simulink model "fir_32tap_8cores"  (R2019b)
settings: Solver=VariableStepAuto  StartTime=0.0  StopTime=T/2  RelTol=1e-3
InitFcn:
  | xmcCheckSlxPath(bdroot)
  | setup
StopFcn:
  | %compare
values from neighbouring files (symbols this model uses):
  c = [30 31 28 29 26 27 24 25 22 23 20 21 18 19 16 17      14 15 12 13 10 11 8 9 6 7 4 5 2 3 0 1]    [setup.m]
undefined symbols (not defined in the file or in its folder): xc7vx485tffg1157
libraries: dspsrcs4 x15, ModelComposer x10, dspsigops x4
settings Model: Creator=abehbood  LastModifiedBy=abehbood
settings SFSimCC: CustomCodeUndefinedFunction=UseInterfaceOnly

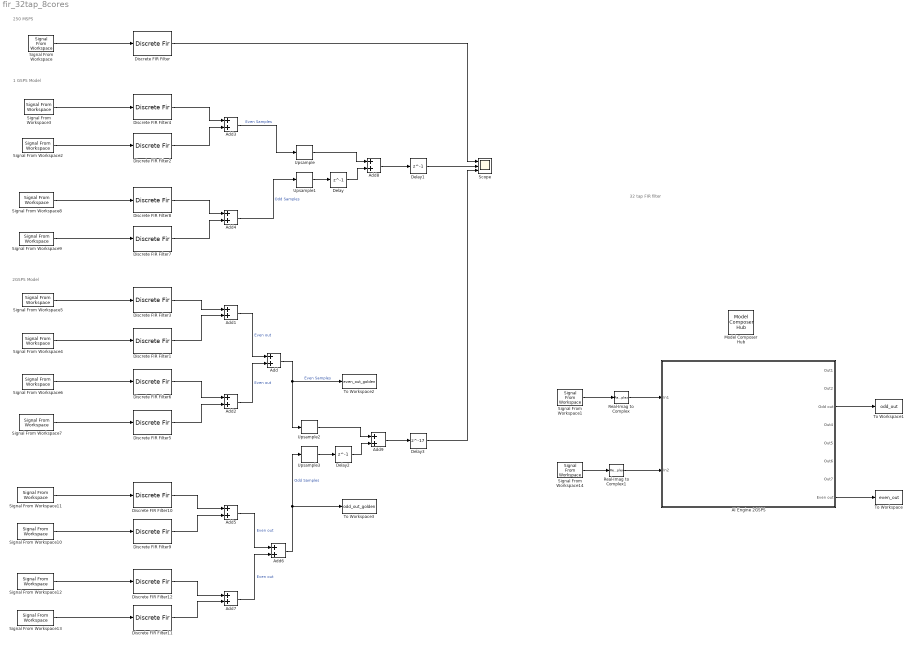
== system fir_32tap_8cores ==
  note: 32 tap FIR filter
  note: 250 MSPS
  note: 2GSPS Model
  note: 1 GSPS Model
  AI Engine 2GSPS : Subsystem
  Add{,1..9} (10 alike) : Sum
  Delay : Delay  DelayLength=1
  Delay1 : Delay  DelayLength=1
  Delay2 : Delay  DelayLength=1
  Delay3 : Delay  DelayLength=17
  Discrete FIR Filter : DiscreteFir  Coefficients=c  InputProcessing=Columns as channels (frame based)  CoefDataTypeStr=int16  ProductDataTypeStr=fixdt(1,48,0)  AccumDataTypeStr=fixdt(1,48,0)  OutDataTypeStr=int16
  Discrete FIR Filter1 : DiscreteFir  Coefficients=c(1:2:32/2)  InputProcessing=Columns as channels (frame based)  CoefDataTypeStr=int16  OutDataTypeStr=int16
  Discrete FIR Filter10 : DiscreteFir  Coefficients=c(32/2+1:2:end)  InputProcessing=Columns as channels (frame based)  CoefDataTypeStr=int16  OutDataTypeStr=int16
  Discrete FIR Filter11 : DiscreteFir  Coefficients=c(2:2:32/2)  InputProcessing=Columns as channels (frame based)  CoefDataTypeStr=int16  OutDataTypeStr=int16
  Discrete FIR Filter12 : DiscreteFir  Coefficients=c(32/2+2:2:end)  InputProcessing=Columns as channels (frame based)  CoefDataTypeStr=int16  OutDataTypeStr=int16
  Discrete FIR Filter2 : DiscreteFir  Coefficients=c(2:2:end)  InputProcessing=Columns as channels (frame based)  CoefDataTypeStr=int16  OutDataTypeStr=int16
  Discrete FIR Filter3 : DiscreteFir  Coefficients=c(32/2+1:2:end)  InputProcessing=Columns as channels (frame based)  CoefDataTypeStr=int16  OutDataTypeStr=int16
  Discrete FIR Filter4 : DiscreteFir  Coefficients=c(1:2:end)  InputProcessing=Columns as channels (frame based)  CoefDataTypeStr=int16  OutDataTypeStr=int16
  Discrete FIR Filter5 : DiscreteFir  Coefficients=c(2:2:32/2)  InputProcessing=Columns as channels (frame based)  CoefDataTypeStr=int16  OutDataTypeStr=int16
  Discrete FIR Filter6 : DiscreteFir  Coefficients=c(32/2+2:2:end)  InputProcessing=Columns as channels (frame based)  CoefDataTypeStr=int16  OutDataTypeStr=int16
  Discrete FIR Filter7 : DiscreteFir  Coefficients=c(2:2:end)  InputProcessing=Columns as channels (frame based)  CoefDataTypeStr=int16  OutDataTypeStr=int16
  Discrete FIR Filter8 : DiscreteFir  Coefficients=c(1:2:end)  InputProcessing=Columns as channels (frame based)  CoefDataTypeStr=int16  OutDataTypeStr=int16
  Discrete FIR Filter9 : DiscreteFir  Coefficients=c(1:2:32/2)  InputProcessing=Columns as channels (frame based)  CoefDataTypeStr=int16  OutDataTypeStr=int16
  Model Composer Hub : ModelComposer/Model Composer Hub  CodeGeneration=off  TargetDirectory=./code  SubsystemName=AI Engine 2GSPS  ExportType=AI Engines  IpVendor=xilinx.com  IpLibrary=hls  IpVersion=1.0  IpHWLanguage=Verilog  CreateTestbench=on  TestbenchStackSize=10  AieCompilerOptions={}  RunAieSim=on  LaunchVitisAnalyzer=off  AieSimTimeout=50000  RunX86Sim=off  X86SimTimeout=10  ProjDevice=xc7vx485tffg1157-1  ProjDevicePart=xc7vx485tffg1157-1  SamplePeriod=-1  ClockFrequency=200  DataPathParallelism=1
  Real-Imag to Complex : RealImagToComplex  Input=Real
  Real-Imag to Complex1 : RealImagToComplex  Input=Real
  Scope : Scope  NumInputPorts=3
  Signal From Workspace : dspsrcs4/Signal From Workspace  X=in  Ts=.5  nsamps=1  OutputAfterFinalValue=Setting to zero  ignoreOrWarnInputAndFrameLengths=off  OutputFrames=off
  Signal From Workspace{1,3,5,9,12} (5 alike) : dspsrcs4/Signal From Workspace  X=in_odd  Ts=1  nsamps=1  OutputAfterFinalValue=Setting to zero  ignoreOrWarnInputAndFrameLengths=off  OutputFrames=off
  Signal From Workspace10 : dspsrcs4/Signal From Workspace  X=in_even_skip_9  Ts=1  nsamps=1  OutputAfterFinalValue=Setting to zero  ignoreOrWarnInputAndFrameLengths=off  OutputFrames=off
  Signal From Workspace11 : dspsrcs4/Signal From Workspace  X=in_even_skip_1  Ts=1  nsamps=1  OutputAfterFinalValue=Setting to zero  ignoreOrWarnInputAndFrameLengths=off  OutputFrames=off
  Signal From Workspace13 : dspsrcs4/Signal From Workspace  X=in_odd_skip_8  Ts=1  nsamps=1  OutputAfterFinalValue=Setting to zero  ignoreOrWarnInputAndFrameLengths=off  OutputFrames=off
  Signal From Workspace14 : dspsrcs4/Signal From Workspace  X=in_even  Ts=1  nsamps=1  OutputAfterFinalValue=Setting to zero  ignoreOrWarnInputAndFrameLengths=off  OutputFrames=off
  Signal From Workspace2 : dspsrcs4/Signal From Workspace  X=in_even  Ts=1  nsamps=1  OutputAfterFinalValue=Setting to zero  ignoreOrWarnInputAndFrameLengths=off  OutputFrames=off
  Signal From Workspace4 : dspsrcs4/Signal From Workspace  X=in_odd_skip_8  Ts=1  nsamps=1  OutputAfterFinalValue=Setting to zero  ignoreOrWarnInputAndFrameLengths=off  OutputFrames=off
  Signal From Workspace6 : dspsrcs4/Signal From Workspace  X=in_even  Ts=1  nsamps=1  OutputAfterFinalValue=Setting to zero  ignoreOrWarnInputAndFrameLengths=off  OutputFrames=off
  Signal From Workspace7 : dspsrcs4/Signal From Workspace  X=in_even_skip_8  Ts=1  nsamps=1  OutputAfterFinalValue=Setting to zero  ignoreOrWarnInputAndFrameLengths=off  OutputFrames=off
  Signal From Workspace8 : dspsrcs4/Signal From Workspace  X=in_even_skip_1  Ts=1  nsamps=1  OutputAfterFinalValue=Setting to zero  ignoreOrWarnInputAndFrameLengths=off  OutputFrames=off
  To Workspace : ToWorkspace  VariableName=even_out  SaveFormat=Structure  SampleTime=-1
  To Workspace1 : ToWorkspace  VariableName=odd_out  SaveFormat=Structure  SampleTime=-1
  To Workspace2 : ToWorkspace  VariableName=even_out_golden  SampleTime=-1
  To Workspace3 : ToWorkspace  VariableName=odd_out_golden  SampleTime=-1
  Upsample{,1..3} (4 alike) : dspsigops/Upsample  N=2  phase=0  InputProcessing=Columns as channels (frame based)  RateOptions=Allow multirate processing  ic=0  mode=Unused parameter value
  wires:
  Signal From Workspace3/1 -> Discrete FIR Filter4/1
  Signal From Workspace2/1 -> Discrete FIR Filter2/1
  Add1/1 -> Add/1  "Even out"
  Discrete FIR Filter4/1 -> Add3/1
  Signal From Workspace4/1 -> Discrete FIR Filter1/1
  Signal From Workspace5/1 -> Discrete FIR Filter3/1
  Signal From Workspace6/1 -> Discrete FIR Filter6/1
  Signal From Workspace7/1 -> Discrete FIR Filter5/1
  Discrete FIR Filter5/1 -> Add2/2
  Discrete FIR Filter6/1 -> Add2/1
  Add2/1 -> Add/2  "Even out"
  Discrete FIR Filter2/1 -> Add3/2
  Add3/1 -> Upsample/1  "Even Samples"
  Discrete FIR Filter8/1 -> Add4/1
  Add4/1 -> Upsample1/1  "Odd Samples"
  Discrete FIR Filter7/1 -> Add4/2
  Signal From Workspace8/1 -> Discrete FIR Filter8/1
  Signal From Workspace9/1 -> Discrete FIR Filter7/1
  Discrete FIR Filter12/1 -> Add7/1
  Signal From Workspace12/1 -> Discrete FIR Filter12/1
  Discrete FIR Filter11/1 -> Add7/2
  Add5/1 -> Add6/1  "Even out"
  Signal From Workspace13/1 -> Discrete FIR Filter11/1
  Discrete FIR Filter9/1 -> Add5/2
  Signal From Workspace10/1 -> Discrete FIR Filter9/1
  Add7/1 -> Add6/2  "Even out"
  Signal From Workspace11/1 -> Discrete FIR Filter10/1
  Discrete FIR Filter10/1 -> Add5/1
  Discrete FIR Filter3/1 -> Add1/1
  Discrete FIR Filter1/1 -> Add1/2
  Upsample1/1 -> Delay/1
  Upsample/1 -> Add8/1
  Delay/1 -> Add8/2
  Add8/1 -> Delay1/1
  Delay1/1 -> Scope/2
  Upsample3/1 -> Delay2/1
  Add6/1 -> To Workspace3/1, Upsample3/1  "Odd Samples"
  Upsample2/1 -> Add9/1
  Delay2/1 -> Add9/2
  Add/1 -> To Workspace2/1, Upsample2/1  "Even Samples"
  Discrete FIR Filter/1 -> Scope/1
  Add9/1 -> Delay3/1
  Delay3/1 -> Scope/3
  Signal From Workspace/1 -> Discrete FIR Filter/1
  Signal From Workspace1/1 -> Real-Imag to Complex/1
  Signal From Workspace14/1 -> Real-Imag to Complex1/1
  Real-Imag to Complex/1 -> AI Engine 2GSPS/1(In1)
  Real-Imag to Complex1/1 -> AI Engine 2GSPS/2(In2)
  AI Engine 2GSPS/8(Even out) -> To Workspace/1
  AI Engine 2GSPS/3(Odd out) -> To Workspace1/1

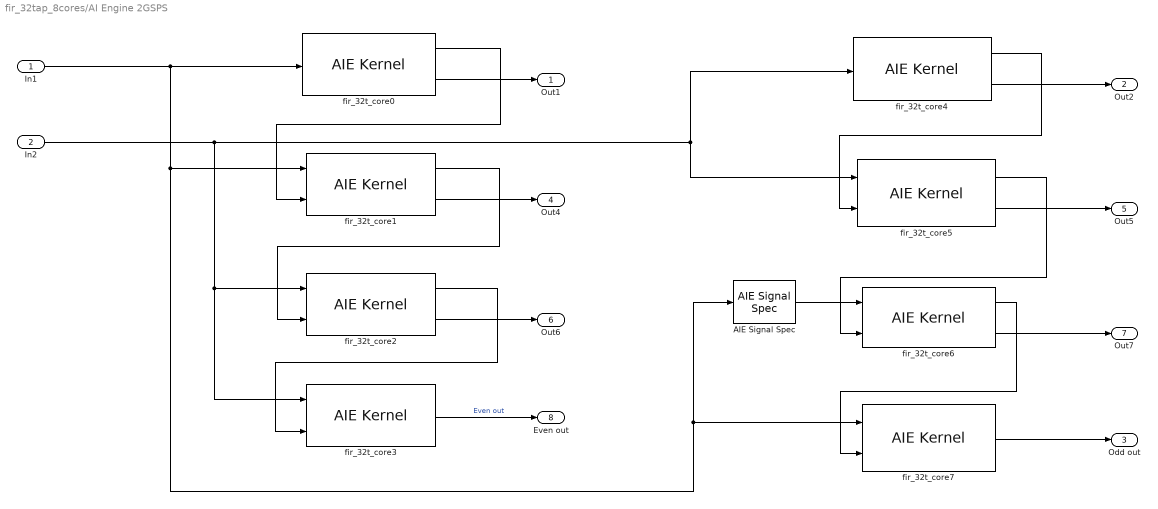
== system fir_32tap_8cores/AI Engine 2GSPS ==
  In1 : Inport
  In2 : Inport  Port=2
  AIE Signal Spec : ModelComposer/AIE Signal Spec  DestFifoDepth=1  SrcFifoDepth=0  PlioWidth=NA
  fir_32t_core0 : ModelComposer/AIE Kernel  PortAttributesTable={'Input', 'sig_in', 'input_stream_cint16 *', '', '', '', '';'Output', 'cascadeout', 'output_stream_cacc48 *', '', '', '', '1';'Output', 'data_out', 'output_stream_cint16 *', '', '', '', '1'}  PortAttributesEnablement={'off', 'off', 'off', 'off', 'off', 'off', 'off';'off', 'off', 'off', 'off', 'off', 'off', 'on';'off', 'off', 'off', 'off', 'off', 'off', 'on'}  FormalArgDecls={'input_stream_cint16 * sig_in', 'output_stream_cacc48 * cascadeout', 'output_stream_cint16 * data_out'}  PortWindowSizes={0.000000000000000000e+00, 0.000000000000000000e+00, 0.000000000000000000e+00}  PortWindowMargins={0.000000000000000000e+00, 0.000000000000000000e+00, 0.000000000000000000e+00}  PortSynchronicities={'sync', 'sync', 'sync'}  PortSignalSizes={0.000000000000000000e+00, 1.000000000000000000e+00, 1.000000000000000000e+00}  SimLibPath=''  FunctionTabVisible=on  FunctionDescription=void fir_32t_core0(input_stream_cint16 * sig_in, output_stream_cacc48 * cascadeout, output_stream_cint16 * data_out)  KernelHeaderFile=src/kernels/inc/fir_32t_core0.h  KernelFunction=fir_32t_core0  KernelFunctionSelect=<empty>  KernelInitFunction=fir_32t_core0_init  KernelSourceFile=fir_32t_core0.cc  KernelSearchPaths={'./data', './src', './src/include', './src/kernels/inc', './src/kernels/src_template'}  PreProcOptions={}  CoreRuntimeRatio=0.9
  fir_32t_core1 : ModelComposer/AIE Kernel  PortAttributesTable={'Input', 'sign_in', 'input_stream_cint16 *', '', '', '', '';'Input', 'cascadein', 'input_stream_cacc48 *', '', '', '', '';'Output', 'cascadeout', 'output_stream_cacc48 *', '', '', '', '1';'Output', 'data_out', 'output_stream_cint16 *', '', '', '', '1'}  PortAttributesEnablement={'off', 'off', 'off', 'off', 'off', 'off', 'off';'off', 'off', 'off', 'off', 'off', 'off', 'off';'off', 'off', 'off', 'off', 'off', 'off', 'on';'off', 'off', 'off', 'off', 'off', 'off', 'on'}  FormalArgDecls={'input_stream_cint16 * sign_in', 'input_stream_cacc48 * cascadein', 'output_stream_cacc48 * cascadeout', 'output_stream_cint16 * data_out'}  PortWindowSizes={0.000000000000000000e+00, 0.000000000000000000e+00, 0.000000000000000000e+00, 0.000000000000000000e+00}  PortWindowMargins={0.000000000000000000e+00, 0.000000000000000000e+00, 0.000000000000000000e+00, 0.000000000000000000e+00}  PortSynchronicities={'sync', 'sync', 'sync', 'sync'}  PortSignalSizes={0.000000000000000000e+00, 0.000000000000000000e+00, 1.000000000000000000e+00, 1.000000000000000000e+00}  SimLibPath=''  FunctionTabVisible=on  FunctionDescription=void fir_32t_core1(input_stream_cint16 * sign_in, input_stream_cacc48 * cascadein, output_stream_cacc48 * cascadeout, output_stream_cint16 * data_out)  KernelHeaderFile=src/kernels/inc/fir_32t_core1.h  KernelFunction=fir_32t_core1  KernelFunctionSelect=<empty>  KernelInitFunction=fir_32t_core1_init  KernelSourceFile=fir_32t_core1.cc  KernelSearchPaths={'./data', './src', './src/include', './src/kernels/inc', './src/kernels/src_template'}  PreProcOptions={}  CoreRuntimeRatio=0.9
  fir_32t_core2 : ModelComposer/AIE Kernel  PortAttributesTable={'Input', 'sign_in', 'input_stream_cint16 *', '', '', '', '';'Input', 'cascadein', 'input_stream_cacc48 *', '', '', '', '';'Output', 'cascadeout', 'output_stream_cacc48 *', '', '', '', '1';'Output', 'data_out', 'output_stream_cint16 *', '', '', '', '1'}  PortAttributesEnablement={'off', 'off', 'off', 'off', 'off', 'off', 'off';'off', 'off', 'off', 'off', 'off', 'off', 'off';'off', 'off', 'off', 'off', 'off', 'off', 'on';'off', 'off', 'off', 'off', 'off', 'off', 'on'}  FormalArgDecls={'input_stream_cint16 * sign_in', 'input_stream_cacc48 * cascadein', 'output_stream_cacc48 * cascadeout', 'output_stream_cint16 * data_out'}  PortWindowSizes={0.000000000000000000e+00, 0.000000000000000000e+00, 0.000000000000000000e+00, 0.000000000000000000e+00}  PortWindowMargins={0.000000000000000000e+00, 0.000000000000000000e+00, 0.000000000000000000e+00, 0.000000000000000000e+00}  PortSynchronicities={'sync', 'sync', 'sync', 'sync'}  PortSignalSizes={0.000000000000000000e+00, 0.000000000000000000e+00, 1.000000000000000000e+00, 1.000000000000000000e+00}  SimLibPath=''  FunctionTabVisible=on  FunctionDescription=void fir_32t_core2(input_stream_cint16 * sign_in, input_stream_cacc48 * cascadein, output_stream_cacc48 * cascadeout, output_stream_cint16 * data_out)  KernelHeaderFile=src/kernels/inc/fir_32t_core2.h  KernelFunction=fir_32t_core2  KernelFunctionSelect=<empty>  KernelInitFunction=fir_32t_core2_init  KernelSourceFile=fir_32t_core2.cc  KernelSearchPaths={'./data', './src', './src/include', './src/kernels/inc', './src/kernels/src_template'}  PreProcOptions={}  CoreRuntimeRatio=0.9
  fir_32t_core3 : ModelComposer/AIE Kernel  PortAttributesTable={'Input', 'sign_in', 'input_stream_cint16 *', '', '', '', '';'Input', 'cascadein', 'input_stream_cacc48 *', '', '', '', '';'Output', 'data_out', 'output_stream_cint16 *', '', '', '', '1'}  PortAttributesEnablement={'off', 'off', 'off', 'off', 'off', 'off', 'off';'off', 'off', 'off', 'off', 'off', 'off', 'off';'off', 'off', 'off', 'off', 'off', 'off', 'on'}  FormalArgDecls={'input_stream_cint16 * sign_in', 'input_stream_cacc48 * cascadein', 'output_stream_cint16 * data_out'}  PortWindowSizes={0.000000000000000000e+00, 0.000000000000000000e+00, 0.000000000000000000e+00}  PortWindowMargins={0.000000000000000000e+00, 0.000000000000000000e+00, 0.000000000000000000e+00}  PortSynchronicities={'sync', 'sync', 'sync'}  PortSignalSizes={0.000000000000000000e+00, 0.000000000000000000e+00, 1.000000000000000000e+00}  SimLibPath=''  FunctionTabVisible=on  FunctionDescription=void fir_32t_core3(input_stream_cint16 * sign_in, input_stream_cacc48 * cascadein, output_stream_cint16 * data_out)  KernelHeaderFile=src/kernels/inc/fir_32t_core3.h  KernelFunction=fir_32t_core3  KernelFunctionSelect=<empty>  KernelInitFunction=fir_32t_core3_init  KernelSourceFile=fir_32t_core3.cc  KernelSearchPaths={'./data', './src', './src/include', './src/kernels/inc', './src/kernels/src_template'}  PreProcOptions={}  CoreRuntimeRatio=0.9
  fir_32t_core4 : ModelComposer/AIE Kernel  PortAttributesTable={'Input', 'sig_in', 'input_stream_cint16 *', '', '', '', '';'Output', 'cascadeout', 'output_stream_cacc48 *', '', '', '', '1';'Output', 'data_out', 'output_stream_cint16 *', '', '', '', '1'}  PortAttributesEnablement={'off', 'off', 'off', 'off', 'off', 'off', 'off';'off', 'off', 'off', 'off', 'off', 'off', 'on';'off', 'off', 'off', 'off', 'off', 'off', 'on'}  FormalArgDecls={'input_stream_cint16 * sig_in', 'output_stream_cacc48 * cascadeout', 'output_stream_cint16 * data_out'}  PortWindowSizes={0.000000000000000000e+00, 0.000000000000000000e+00, 0.000000000000000000e+00}  PortWindowMargins={0.000000000000000000e+00, 0.000000000000000000e+00, 0.000000000000000000e+00}  PortSynchronicities={'sync', 'sync', 'sync'}  PortSignalSizes={0.000000000000000000e+00, 1.000000000000000000e+00, 1.000000000000000000e+00}  SimLibPath=''  FunctionTabVisible=on  FunctionDescription=void fir_32t_core4(input_stream_cint16 * sig_in, output_stream_cacc48 * cascadeout, output_stream_cint16 * data_out)  KernelHeaderFile=src/kernels/inc/fir_32t_core4.h  KernelFunction=fir_32t_core4  KernelFunctionSelect=<empty>  KernelInitFunction=fir_32t_core4_init  KernelSourceFile=fir_32t_core4.cc  KernelSearchPaths={'./data', './src', './src/include', './src/kernels/inc', './src/kernels/src_template'}  PreProcOptions={}  CoreRuntimeRatio=0.9
  fir_32t_core5 : ModelComposer/AIE Kernel  PortAttributesTable={'Input', 'sign_in', 'input_stream_cint16 *', '', '', '', '';'Input', 'cascadein', 'input_stream_cacc48 *', '', '', '', '';'Output', 'cascadeout', 'output_stream_cacc48 *', '', '', '', '1';'Output', 'data_out', 'output_stream_cint16 *', '', '', '', '1'}  PortAttributesEnablement={'off', 'off', 'off', 'off', 'off', 'off', 'off';'off', 'off', 'off', 'off', 'off', 'off', 'off';'off', 'off', 'off', 'off', 'off', 'off', 'on';'off', 'off', 'off', 'off', 'off', 'off', 'on'}  FormalArgDecls={'input_stream_cint16 * sign_in', 'input_stream_cacc48 * cascadein', 'output_stream_cacc48 * cascadeout', 'output_stream_cint16 * data_out'}  PortWindowSizes={0.000000000000000000e+00, 0.000000000000000000e+00, 0.000000000000000000e+00, 0.000000000000000000e+00}  PortWindowMargins={0.000000000000000000e+00, 0.000000000000000000e+00, 0.000000000000000000e+00, 0.000000000000000000e+00}  PortSynchronicities={'sync', 'sync', 'sync', 'sync'}  PortSignalSizes={0.000000000000000000e+00, 0.000000000000000000e+00, 1.000000000000000000e+00, 1.000000000000000000e+00}  SimLibPath=''  FunctionTabVisible=on  FunctionDescription=void fir_32t_core5(input_stream_cint16 * sign_in, input_stream_cacc48 * cascadein, output_stream_cacc48 * cascadeout, output_stream_cint16 * data_out)  KernelHeaderFile=src/kernels/inc/fir_32t_core5.h  KernelFunction=fir_32t_core5  KernelFunctionSelect=<empty>  KernelInitFunction=fir_32t_core5_init  KernelSourceFile=fir_32t_core5.cc  KernelSearchPaths={'./data', './src', './src/include', './src/kernels/inc', './src/kernels/src_template'}  PreProcOptions={}  CoreRuntimeRatio=0.9
  fir_32t_core6 : ModelComposer/AIE Kernel  PortAttributesTable={'Input', 'sign_in', 'input_stream_cint16 *', '', '', '', '';'Input', 'cascadein', 'input_stream_cacc48 *', '', '', '', '';'Output', 'cascadeout', 'output_stream_cacc48 *', '', '', '', '1';'Output', 'data_out', 'output_stream_cint16 *', '', '', '', '1'}  PortAttributesEnablement={'off', 'off', 'off', 'off', 'off', 'off', 'off';'off', 'off', 'off', 'off', 'off', 'off', 'off';'off', 'off', 'off', 'off', 'off', 'off', 'on';'off', 'off', 'off', 'off', 'off', 'off', 'on'}  FormalArgDecls={'input_stream_cint16 * sign_in', 'input_stream_cacc48 * cascadein', 'output_stream_cacc48 * cascadeout', 'output_stream_cint16 * data_out'}  PortWindowSizes={0.000000000000000000e+00, 0.000000000000000000e+00, 0.000000000000000000e+00, 0.000000000000000000e+00}  PortWindowMargins={0.000000000000000000e+00, 0.000000000000000000e+00, 0.000000000000000000e+00, 0.000000000000000000e+00}  PortSynchronicities={'sync', 'sync', 'sync', 'sync'}  PortSignalSizes={0.000000000000000000e+00, 0.000000000000000000e+00, 1.000000000000000000e+00, 1.000000000000000000e+00}  SimLibPath=''  FunctionTabVisible=on  FunctionDescription=void fir_32t_core6(input_stream_cint16 * sign_in, input_stream_cacc48 * cascadein, output_stream_cacc48 * cascadeout, output_stream_cint16 * data_out)  KernelHeaderFile=src/kernels/inc/fir_32t_core6.h  KernelFunction=fir_32t_core6  KernelFunctionSelect=<empty>  KernelInitFunction=fir_32t_core6_init  KernelSourceFile=fir_32t_core6.cc  KernelSearchPaths={'./data', './src', './src/include', './src/kernels/inc', './src/kernels/src_template'}  PreProcOptions={}  CoreRuntimeRatio=0.9
  fir_32t_core7 : ModelComposer/AIE Kernel  PortAttributesTable={'Input', 'sign_in', 'input_stream_cint16 *', '', '', '', '';'Input', 'cascadein', 'input_stream_cacc48 *', '', '', '', '';'Output', 'data_out', 'output_stream_cint16 *', '', '', '', '1'}  PortAttributesEnablement={'off', 'off', 'off', 'off', 'off', 'off', 'off';'off', 'off', 'off', 'off', 'off', 'off', 'off';'off', 'off', 'off', 'off', 'off', 'off', 'on'}  FormalArgDecls={'input_stream_cint16 * sign_in', 'input_stream_cacc48 * cascadein', 'output_stream_cint16 * data_out'}  PortWindowSizes={0.000000000000000000e+00, 0.000000000000000000e+00, 0.000000000000000000e+00}  PortWindowMargins={0.000000000000000000e+00, 0.000000000000000000e+00, 0.000000000000000000e+00}  PortSynchronicities={'sync', 'sync', 'sync'}  PortSignalSizes={0.000000000000000000e+00, 0.000000000000000000e+00, 1.000000000000000000e+00}  SimLibPath=''  FunctionTabVisible=on  FunctionDescription=void fir_32t_core7(input_stream_cint16 * sign_in, input_stream_cacc48 * cascadein, output_stream_cint16 * data_out)  KernelHeaderFile=src/kernels/inc/fir_32t_core7.h  KernelFunction=fir_32t_core7  KernelFunctionSelect=<empty>  KernelInitFunction=fir_32t_core7_init  KernelSourceFile=fir_32t_core7.cc  KernelSearchPaths={'./data', './src', './src/include', './src/kernels/inc', './src/kernels/src_template'}  PreProcOptions={}  CoreRuntimeRatio=0.9
  Out1 : Outport  VectorParamsAs1DForOutWhenUnconnected=off
  Out2 : Outport  Port=2  VectorParamsAs1DForOutWhenUnconnected=off
  Odd out : Outport  Port=3  VectorParamsAs1DForOutWhenUnconnected=off
  Out4 : Outport  Port=4  VectorParamsAs1DForOutWhenUnconnected=off
  Out5 : Outport  Port=5  VectorParamsAs1DForOutWhenUnconnected=off
  Out6 : Outport  Port=6  VectorParamsAs1DForOutWhenUnconnected=off
  Out7 : Outport  Port=7  VectorParamsAs1DForOutWhenUnconnected=off
  Even out : Outport  Port=8  VectorParamsAs1DForOutWhenUnconnected=off
  wires:
  fir_32t_core6/2 -> Out7/1
  fir_32t_core1/2 -> Out4/1
  fir_32t_core0/1 -> fir_32t_core1/2
  fir_32t_core4/2 -> Out2/1
  fir_32t_core3/1 -> Even out/1  "Even out"
  fir_32t_core5/2 -> Out5/1
  fir_32t_core2/2 -> Out6/1
  fir_32t_core7/1 -> Odd out/1
  fir_32t_core1/1 -> fir_32t_core2/2
  fir_32t_core4/1 -> fir_32t_core5/2
  fir_32t_core6/1 -> fir_32t_core7/2
  fir_32t_core0/2 -> Out1/1
  fir_32t_core2/1 -> fir_32t_core3/2
  fir_32t_core5/1 -> fir_32t_core6/2
  In2/1 -> fir_32t_core3/1, fir_32t_core2/1, fir_32t_core5/1, fir_32t_core4/1
  AIE Signal Spec/1 -> fir_32t_core6/1
  In1/1 -> AIE Signal Spec/1, fir_32t_core7/1, fir_32t_core1/1, fir_32t_core0/1
